simulink model "Realistic_scheme"  (R2020b)
settings: Solver=VariableStepAuto  StartTime=0.0  StopTime=10  RelTol=1e-3
values from neighbouring files (symbols this model uses):
  A = [[0 0 1 0] ... (first row only)    [Inverted_pendulum.m]
  B = [0 ... (first row only)    [Inverted_pendulum.m]
  C = [[1 0 0 0] ... (first row only)    [Inverted_pendulum.m]
  D = 0    [Inverted_pendulum.m]
undefined symbols (not defined in the file or in its folder): Con_from_V, Con_to_V, K, Ts, V_max_in, V_max_out, wc
settings Model: Creator=elina  LastModifiedBy=gebruiker

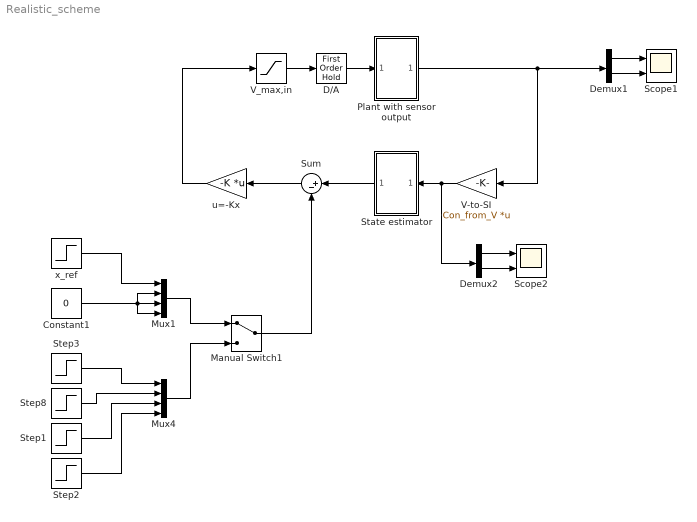
== system Realistic_scheme ==
  Constant1 : Constant  Value=0
  D/A : FirstOrderHold  OutputAlgorithm=Fast (Minimize Error)  ErrorTolerance=inf
  Demux1 : Demux  Outputs=2
  Demux2 : Demux  Outputs=2
  Manual Switch1 : ManualSwitch
  Mux1 : Mux
  Mux4 : Mux
  Plant with sensor output : Subsystem
  Scope1 : Scope  NumInputPorts=2
  Scope2 : Scope  NumInputPorts=2
  State estimator : Subsystem
  Step1 : Step  Time=0  After=0  SampleTime=0
  Step2 : Step  After=0  SampleTime=0
  Step3 : Step  Time=0  After=0.15  SampleTime=0
  Step8 : Step  After=0  SampleTime=0
  Sum : Sum  Inputs=|+-
  V-to-SI : Gain  Gain=Con_from_V  Multiplication=Matrix(K*u)
  V_max,in : Saturate  UpperLimit=V_max_in  LowerLimit=-V_max_in
  u=-Kx : Gain  Gain=-K  Multiplication=Matrix(K*u)
  x_ref : Step  Time=0  After=0.05  SampleTime=0
  wires:
  x_ref/1 -> Mux1/1
  Constant1/1 -> Mux1/2, Mux1/4, Mux1/3
  State estimator/1(Out1) -> Sum/1
  Sum/1 -> u=-Kx/1
  u=-Kx/1 -> V_max,in/1
  V_max,in/1 -> D/A/1
  V-to-SI/1 -> Demux2/1, State estimator/1(In1)
  Plant with sensor output/1(Out1) -> V-to-SI/1, Demux1/1
  Mux1/1 -> Manual Switch1/1
  Mux4/1 -> Manual Switch1/2
  Step1/1 -> Mux4/3
  Step2/1 -> Mux4/4
  Step8/1 -> Mux4/2
  Step3/1 -> Mux4/1
  Manual Switch1/1 -> Sum/2
  D/A/1 -> Plant with sensor output/1(In1)
  Demux1/1 -> Scope1/1
  Demux1/2 -> Scope1/2
  Demux2/1 -> Scope2/1
  Demux2/2 -> Scope2/2

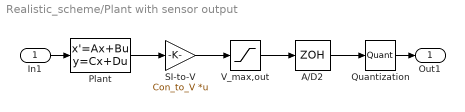
== system Realistic_scheme/Plant with sensor output ==
  In1 : Inport
  A/D2 : ZeroOrderHold  SampleTime=Ts
  Plant : StateSpace  A=A  B=B  C=C  D=D  InitialCondition=[0, 0, 0, 0]
  Quantization : Quantizer  QuantizationInterval=quant_step
  SI-to-V : Gain  Gain=Con_to_V  Multiplication=Matrix(K*u)
  V_max,out : Saturate  UpperLimit=V_max_out  LowerLimit=-V_max_out
  Out1 : Outport
  wires:
  Plant/1 -> SI-to-V/1
  V_max,out/1 -> A/D2/1
  SI-to-V/1 -> V_max,out/1
  A/D2/1 -> Quantization/1
  In1/1 -> Plant/1
  Quantization/1 -> Out1/1

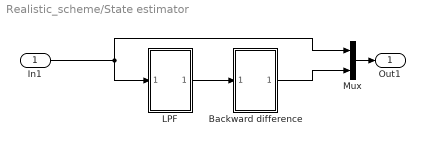
== system Realistic_scheme/State estimator ==
  In1 : Inport
  Backward difference : Subsystem
  LPF : Subsystem
  Mux : Mux  Inputs=2
  Out1 : Outport
  wires:
  LPF/1(Out1) -> Backward difference/1(In1)
  Backward difference/1(Out1) -> Mux/2
  Mux/1 -> Out1/1
  In1/1 -> Mux/1, LPF/1(In1)

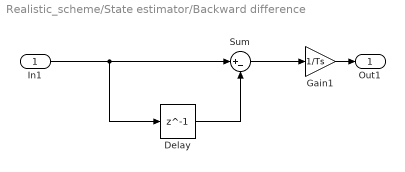
== system Realistic_scheme/State estimator/Backward difference ==
  In1 : Inport
  Delay : Delay  DelayLength=1  InitialCondition=0
  Gain1 : Gain  Gain=1/Ts
  Sum : Sum  Inputs=|+-
  Out1 : Outport
  wires:
  Delay/1 -> Sum/2
  Gain1/1 -> Out1/1
  In1/1 -> Delay/1, Sum/1
  Sum/1 -> Gain1/1

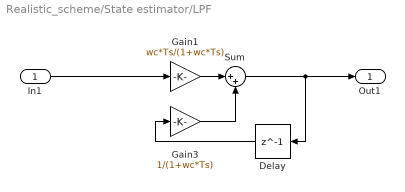
== system Realistic_scheme/State estimator/LPF ==
  In1 : Inport
  Delay : Delay  DelayLength=1
  Gain1 : Gain  Gain=wc*Ts/(1+wc*Ts)
  Gain3 : Gain  Gain=1/(1+wc*Ts)
  Sum : Sum  Inputs=|++
  Out1 : Outport
  wires:
  Gain3/1 -> Sum/2
  Sum/1 -> Out1/1, Delay/1
  Delay/1 -> Gain3/1
  In1/1 -> Gain1/1
  Gain1/1 -> Sum/1
